simulink library "LiCell"  (R2016a)
settings: Solver=ode45  StartTime=0.0  StopTime=10.0  RelTol=1e-3
undefined symbols (not defined in the file or in its folder): Battery
libraries: fl_lib x6, LiBatteryElements_lib x4, nesl_utility x2
settings Model: Creator=jgazzarr  LastModifiedBy=jgazzarr
settings DataIOCC: LimitDataPoints=on  SaveFormat=Array  SignalLoggingSaveFormat=ModelDataLogs
settings OptimizationCC: ExpressionDepthLimit=2147483647
settings DebuggingCC: UnderspecifiedInitializationDetection=Classic  MergeDetectMultiDrivingBlocksExec=none  SolverPrmCheckMsg=warning  FcnCallInpInsideContextMsg=EnableAllAsWarning  StateNameClashWarn=warning
settings HardwareCC: ProdBitPerPointer=32  ProdLargestAtomicFloat=None  ProdIntDivRoundTo=Undefined  ProdEndianess=Unspecified  ProdWordSize=32  ProdHWDeviceType=32-bit Generic
settings ModelReferenceCC: PropagateSignalLabelsOutOfModel=off
settings ConfigComp: CovModelRefEnable=Off  CovSFcnEnable=off

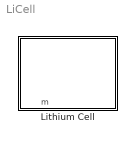
== system LiCell ==
  Lithium Cell : Subsystem  mask{Battery=Battery(1)}
      mask prompts: Battery "Battery Parameter Structure"
      settings: AttributesFormatString=%<Battery>
      mask Display:
      | image(imread('battery.jpg'))
      | color('red')
      | port_label('LConn',1,'H')
      | port_label('LConn',2,'+')
      | port_label('RConn',1,'-')
      | % port_label('LConn',3,'T')
      | % port_label('RConn',2,'SOC')
      | port_label('output',1,'m')

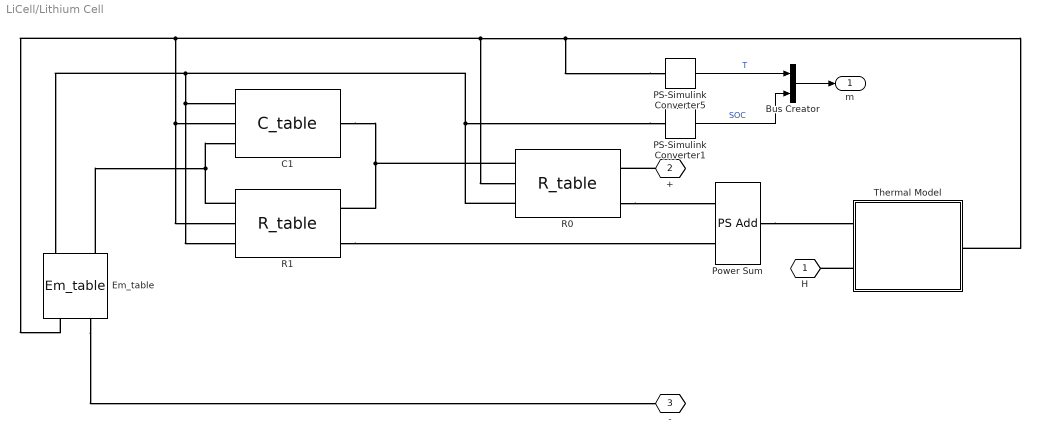
== system LiCell/Lithium Cell ==
  Bus Creator : BusCreator  Inputs=2
  C1 : LiBatteryElements_lib/C_table  C_Table=Battery.C1_LUT F  SOC_Table=Battery.SOC_LUT  Temp_Table=Battery.Temperature_LUT K  v0=0 V  mask(C_table){}
      mask Display: image('C_fig.png')
  Em_table : LiBatteryElements_lib/Em_table  C_Table=Battery.Capacity_LUT hr*A  Em_Table=Battery.Em_LUT V  SOC_Table=Battery.SOC_LUT  Temp_Table=Battery.Temperature_LUT K  Qinit=Battery.Qe_init hr*A  mask(Em_table){}
      mask Display: image('V_fig.png')
  PS-Simulink Converter1 : nesl_utility/PS-Simulink Converter  PhysicalDomain=network_engine_domain  SubClassName=ps_output  LeftPortType=input  RightPortType=output  PseudoPeriodic=off  Frequencies=[]  Unit=1  AffineConversion=off
  PS-Simulink Converter5 : nesl_utility/PS-Simulink Converter  PhysicalDomain=network_engine_domain  SubClassName=ps_output  LeftPortType=input  RightPortType=output  PseudoPeriodic=off  Frequencies=[]  Unit=degC  AffineConversion=on
  Power Sum : fl_lib/Physical Signals/Functions/PS Add
  R0 : LiBatteryElements_lib/R_table  R_Table=Battery.R0_LUT Ohm  SOC_Table=Battery.SOC_LUT  Temp_Table=Battery.Temperature_LUT K  mask(R_table){}
      mask Display: image('R_fig.png')
  R1 : LiBatteryElements_lib/R_table  R_Table=Battery.R1_LUT Ohm  SOC_Table=Battery.SOC_LUT  Temp_Table=Battery.Temperature_LUT K  mask(R_table){}
      mask Display: image('R_fig.png')
  Thermal Model : Subsystem
  H : PMIOPort  Tag=PMCPort  Port=1  Side=Left
  + : PMIOPort  Tag=PMCPort  Port=2  Side=Left
  - : PMIOPort  Tag=PMCPort  Port=3  Side=Right
  m : Outport
  wires:
  PS-Simulink Converter5/1 -> Bus Creator/1  "T"
  PS-Simulink Converter1/1 -> Bus Creator/2  "SOC"
  Bus Creator/1 -> m/1
  connections:
  R0/RConn2 -- Power Sum/LConn1
  R0/LConn1 -- C1/RConn1 -- R1/RConn1
  Power Sum/RConn1 -- Thermal Model/LConn1
  PS-Simulink Converter5/LConn1 -- C1/LConn2 -- R1/LConn2 -- Em_table/RConn2 -- R0/LConn2 -- Thermal Model/RConn1
  R1/RConn2 -- Power Sum/LConn2
  R1/LConn1 -- C1/LConn1 -- Em_table/LConn1
  +/RConn1 -- R0/RConn1
  Em_table/RConn1 -- -/RConn1
  Thermal Model/LConn2 -- H/RConn1
  PS-Simulink Converter1/LConn1 -- C1/LConn3 -- R1/LConn3 -- Em_table/LConn3 -- R0/LConn3

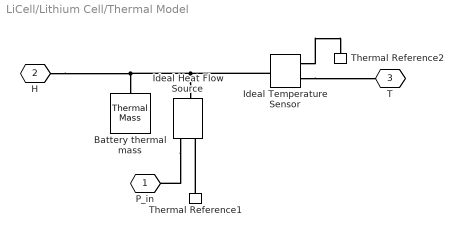
== system LiCell/Lithium Cell/Thermal Model ==
  Battery thermal mass : fl_lib/Thermal/Thermal Elements/Thermal Mass  mass=Battery.cell_mass kg  sp_heat=Battery.cell_Cp_heat J/kg/K  T_specify=on  T_priority=High  T=Battery.T_init K  Q_specify=off  Q_priority=High  Q=0 J/s
  Ideal Temperature Sensor : fl_lib/Thermal/Thermal Sensors/Ideal Temperature Sensor
  Ideal Heat Flow Source : fl_lib/Thermal/Thermal Sources/Ideal Heat Flow Source
  Thermal Reference1 : fl_lib/Thermal/Thermal Elements/Thermal Reference
  Thermal Reference2 : fl_lib/Thermal/Thermal Elements/Thermal Reference
  P_in : PMIOPort  Tag=PMCPort  Port=1  Side=Left
  H : PMIOPort  Tag=PMCPort  Port=2  Side=Left
  T : PMIOPort  Tag=PMCPort  Port=3  Side=Right
  connections:
  Ideal Heat Flow Source/RConn1 -- P_in/RConn1
  Ideal Heat Flow Source/LConn1 -- Battery thermal mass/LConn1 -- H/RConn1 -- Ideal Temperature Sensor/LConn1
  Thermal Reference1/LConn1 -- Ideal Heat Flow Source/RConn2
  Ideal Temperature Sensor/RConn2 -- T/RConn1
  Ideal Temperature Sensor/RConn1 -- Thermal Reference2/LConn1
